simulink model "proc_control_node"  (R2020a)
settings: Solver=FixedStepAuto  StartTime=0.0  StopTime=inf  FixedStep=1/60  RelTol=1e-3
model workspace (MAT data in the model file):
  SL_ROS_VariableLengthArrays_MaxSizes.CommonInfo.ArrayTruncateAction = 'EmitWarning'
  SL_ROS_VariableLengthArrays_MaxSizes.MsgTypeMap = containers.Map
  SL_ROS_VariableLengthArrays_MaxSizes.MsgTypeMap.serialization.keys = {}
  SL_ROS_VariableLengthArrays_MaxSizes.MsgTypeMap.serialization.values = {}
  SL_ROS_VariableLengthArrays_MaxSizes.MsgTypeMap.serialization.uniformity = 0
  SL_ROS_VariableLengthArrays_MaxSizes.MsgTypeMap.serialization.keyType = 'char'
  SL_ROS_VariableLengthArrays_MaxSizes.MsgTypeMap.serialization.valueType = 'any'
undefined symbols (not defined in the file or in its folder): InitAUVPlant, InitController, mpc, physics, simulation
libraries: robotlib x21
settings Model: SimulationMode=accelerator  PauseTimes=1000  EnablePacing=on  Creator=Lamarre  LastModifiedBy=lamarre
settings OptimizationCC: EnhancedBackFolding=on  PassReuseOutputArgsAs=Individual arguments  ZeroExternalMemoryAtStartup=off  ZeroInternalMemoryAtStartup=off  MaxStackSize=64  OptimizeBlockOrder=speed  DifferentSizesBufferReuse=on  OptimizationCustomize=off  EfficientTunableParamExpr=on
settings DebuggingCC: ParameterTunabilityLossMsg=error  FcnCallInpInsideContextMsg=warning  UnderSpecifiedDimensionMsg=warning
settings HardwareCC: ProdBitPerPointer=32  ProdBitPerSizeT=32  ProdBitPerPtrDiffT=32  ProdLargestAtomicInteger=Long  ProdWordSize=32  ProdHWDeviceType=ARM Compatible->ARM 8
settings ModelReferenceCC: ModelReferenceNumInstancesAllowed=Single
settings SFSimCC: MATLABDynamicMemAlloc=off
settings RTWCC: SystemTargetFile=ert.tlc  HardwareBoard=Robot Operating System (ROS)  TemplateMakefile=ert_default_tmf  Toolchain=Catkin  BuildConfiguration=Faster Runs  TargetLang=C++
settings CodeAppCC: ForceParamTrailComments=on  IgnoreCustomStorageClasses=off  OperatorAnnotations=on  SimulinkDataObjDesc=on  SFDataObjDesc=on  InsertBlockDesc=on
settings ERTTargetCC: MultiInstanceERTCode=on  CodeInterfacePackaging=C++ class  SupportContinuousTime=on  SupportVariableSizeSignals=on  MultiInstanceErrorCode=Warning  RootIOFormat=Structure reference

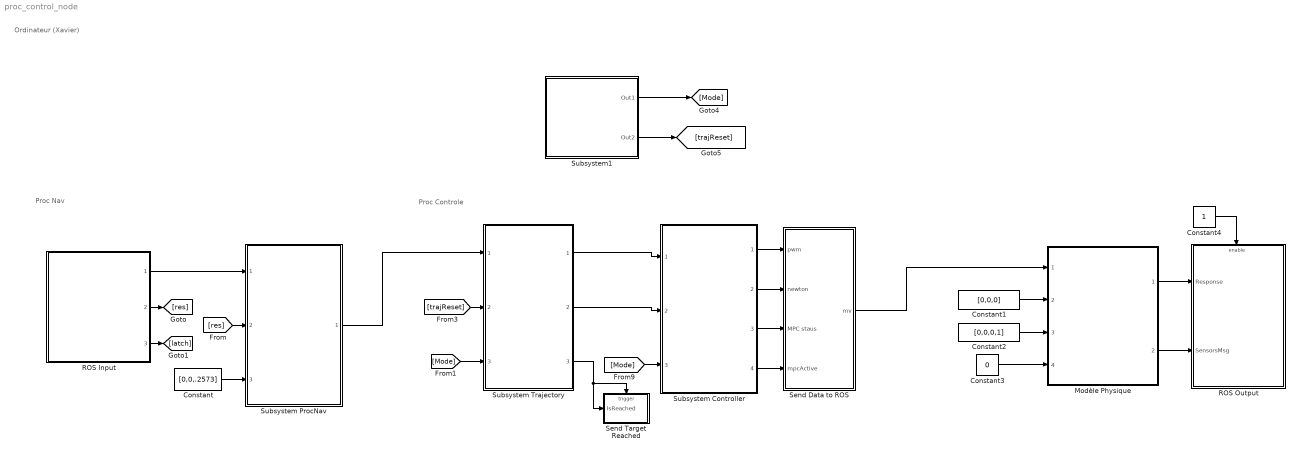
== system proc_control_node ==
  note: Proc Nav
  note: Proc Controle
  note: Ordinateur (Xavier)
  Constant : Constant  Value=[0,0,.2573]
  Constant1 : Constant  Value=[0,0,0]
  Constant2 : Constant  Value=[0,0,0,1]
  Constant3 : Constant  Value=0
  Constant4 : Constant
  Modèle Physique : Subsystem  InitFcn=InitAUVPlant;  ReferencedSubsystem=AUVPlant
  ROS Input : Subsystem  ReferencedSubsystem=proc_nav_ros_input
  ROS Output : Subsystem
  Send Data to ROS : Subsystem
  "Send Target Reached " : Subsystem
  Subsystem Controller : Subsystem  InitFcn=InitController;  ReferencedSubsystem=Controller
  Subsystem ProcNav : Subsystem  ReferencedSubsystem=ProcNav
  Subsystem Trajectory : Subsystem  InitFcn=|  ReferencedSubsystem=Trajectory
      | InitTrajectory
      | %trajec;
  Subsystem1 : Subsystem
  wires:
  Constant/1 -> Subsystem ProcNav/3
  ROS Input/1 -> Subsystem ProcNav/1
  ROS Input/2 -> [res]
  [res] -> Subsystem ProcNav/2
  ROS Input/3 -> [latch]
  [Mode] -> Subsystem Controller/3
  [Mode] -> Subsystem Trajectory/3
  Subsystem Trajectory/1 -> Subsystem Controller/1
  [trajReset] -> Subsystem Trajectory/2
  Subsystem Trajectory/3 -> "Send Target Reached "/1(IsReached), "Send Target Reached "/Trigger
  Subsystem ProcNav/1 -> Subsystem Trajectory/1
  Subsystem Trajectory/2 -> Subsystem Controller/2
  Subsystem1/2(Out2) -> [trajReset]
  Subsystem1/1(Out1) -> [Mode]
  Constant1/1 -> Modèle Physique/2
  Constant2/1 -> Modèle Physique/3
  Constant3/1 -> Modèle Physique/4
  Modèle Physique/1 -> ROS Output/1(Response)
  Modèle Physique/2 -> ROS Output/2(SensorsMsg)
  Constant4/1 -> ROS Output/Enable
  Subsystem Controller/1 -> Send Data to ROS/1(pwm)
  Subsystem Controller/2 -> Send Data to ROS/2(newton)
  Subsystem Controller/3 -> Send Data to ROS/3(MPC staus)
  Subsystem Controller/4 -> Send Data to ROS/4(mpcActive)
  Send Data to ROS/1(mv) -> Modèle Physique/1

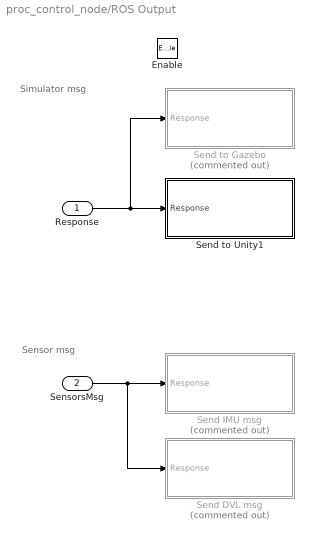
== system proc_control_node/ROS Output ==
  note: Sensor msg
  note: Simulator msg
  Response : Inport
  SensorsMsg : Inport  Port=2
  Enable : EnablePort
  Send DVL msg : Subsystem  Commented=on
  Send IMU msg : Subsystem  Commented=on
  Send to Gazebo : Subsystem  Commented=on  InitFcn=""
  Send to Unity1 : Subsystem
  wires:
  Response/1 -> Send to Unity1/1(Response), Send to Gazebo/1(Response)
  SensorsMsg/1 -> Send DVL msg/1(Response), Send IMU msg/1(Response)

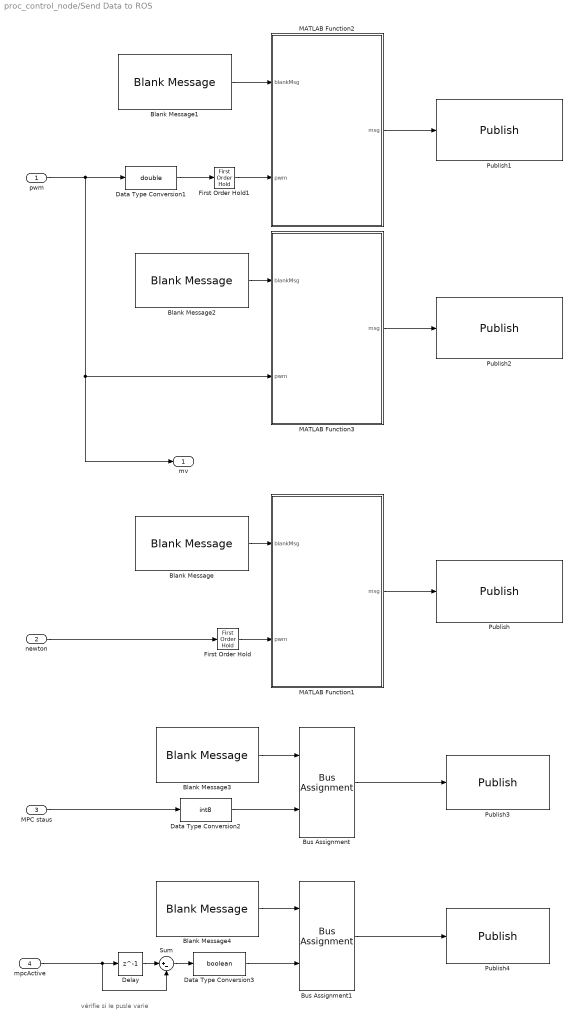
== system proc_control_node/Send Data to ROS ==
  note: vérifie si le pusle varie
  pwm : Inport
  newton : Inport  Port=2
  MPC staus : Inport  Port=3
  mpcActive : Inport  Port=4
  Blank Message : robotlib/Blank Message  messageClass=Message  entityType=std_msgs/Int8MultiArray  messageType=std_msgs/Int8MultiArray  SampleTime=inf
  Blank Message1 : robotlib/Blank Message  messageClass=Message  entityType=std_msgs/UInt16MultiArray  messageType=std_msgs/UInt16MultiArray  SampleTime=inf
  Blank Message2 : robotlib/Blank Message  messageClass=Message  entityType=std_msgs/UInt16MultiArray  messageType=std_msgs/UInt16MultiArray  SampleTime=inf
  Blank Message3 : robotlib/Blank Message  messageClass=Message  entityType=std_msgs/Int8  messageType=std_msgs/Int8  SampleTime=inf
  Blank Message4 : robotlib/Blank Message  messageClass=Message  entityType=std_msgs/Bool  messageType=std_msgs/Bool  SampleTime=-1
  Bus Assignment : BusAssignment  AssignedSignals=Data
  Bus Assignment1 : BusAssignment  AssignedSignals=Data
  Data Type Conversion1 : DataTypeConversion  OutDataTypeStr=double  RndMeth=Nearest
  Data Type Conversion2 : DataTypeConversion  OutDataTypeStr=int8  RndMeth=Nearest
  Data Type Conversion3 : DataTypeConversion  OutDataTypeStr=boolean  RndMeth=Nearest
  Delay : Delay  DelayLength=1  SampleTime=mpc.Ts
  First Order Hold : FirstOrderHold  ErrorTolerance=inf  AllowContinuousInput=on
  First Order Hold1 : FirstOrderHold  ErrorTolerance=inf  AllowContinuousInput=on
  MATLAB Function1 : MATLAB Function  TreatAsAtomicUnit=on  SystemSampleTime=1/30
  MATLAB Function2 : MATLAB Function  TreatAsAtomicUnit=on  SystemSampleTime=1/30
  MATLAB Function3 : MATLAB Function  TreatAsAtomicUnit=on
  Publish : robotlib/Publish  topicSource=Specify your own  topic=/telemetry/thruster_newton  messageType=std_msgs/Int8MultiArray  messageQueueLength=1
  Publish1 : robotlib/Publish  topicSource=Specify your own  topic=/telemetry/thruster_pwm  messageType=std_msgs/UInt16MultiArray  messageQueueLength=1
  Publish2 : robotlib/Publish  topicSource=Specify your own  topic=/provider_thruster/thruster_pwm  messageType=std_msgs/UInt16MultiArray  messageQueueLength=1
  Publish3 : robotlib/Publish  topicSource=Specify your own  topic=proc_control/mpc_status  messageType=std_msgs/Int8  messageQueueLength=1
  Publish4 : robotlib/Publish  topicSource=Specify your own  topic=proc_control/is_mpc_active  messageType=std_msgs/Bool  messageQueueLength=1
  Sum : Sum  Inputs=|+-
  mv : Outport
  wires:
  MATLAB Function1/1(msg) -> Publish/1
  Blank Message/1 -> MATLAB Function1/1(blankMsg)
  First Order Hold/1 -> MATLAB Function1/2(pwm)
  MATLAB Function2/1(msg) -> Publish1/1
  Blank Message1/1 -> MATLAB Function2/1(blankMsg)
  newton/1 -> First Order Hold/1
  Data Type Conversion1/1 -> First Order Hold1/1
  First Order Hold1/1 -> MATLAB Function2/2(pwm)
  MATLAB Function3/1(msg) -> Publish2/1
  pwm/1 -> mv/1, MATLAB Function3/2(pwm), Data Type Conversion1/1
  Blank Message2/1 -> MATLAB Function3/1(blankMsg)
  Blank Message3/1 -> Bus Assignment/1
  Bus Assignment/1 -> Publish3/1
  Data Type Conversion2/1 -> Bus Assignment/2
  MPC staus/1 -> Data Type Conversion2/1
  Data Type Conversion3/1 -> Bus Assignment1/2
  Bus Assignment1/1 -> Publish4/1
  Blank Message4/1 -> Bus Assignment1/1
  mpcActive/1 -> Delay/1, Sum/2
  Delay/1 -> Sum/1
  Sum/1 -> Data Type Conversion3/1

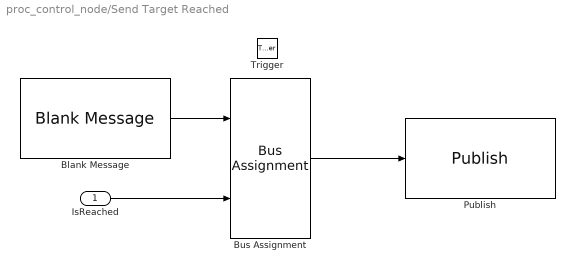
== system proc_control_node/Send Target Reached  ==
  IsReached : Inport
  Trigger : TriggerPort  TriggerType=either  VariantControl=Variant  PortDimensions=1
  Blank Message : robotlib/Blank Message  messageClass=Message  entityType=std_msgs/Bool  messageType=std_msgs/Bool  SampleTime=inf
  Bus Assignment : BusAssignment  AssignedSignals=Data
  Publish : robotlib/Publish  topicSource=Specify your own  topic=proc_control_matlab/target_reached  messageType=std_msgs/Bool  messageQueueLength=1
  wires:
  Blank Message/1 -> Bus Assignment/1
  IsReached/1 -> Bus Assignment/2
  Bus Assignment/1 -> Publish/1

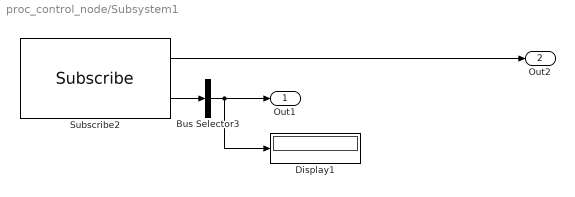
== system proc_control_node/Subsystem1 ==
  Bus Selector3 : BusSelector  OutputSignals=Data  OutputAsBus=on
  Display1 : Display
  Subscribe2 : robotlib/Subscribe  topicSource=Specify your own  topic=/proc_control/set_mode  messageType=std_msgs/UInt8  sampleTime=.25  messageQueueLength=1
  Out1 : Outport
  Out2 : Outport  Port=2
  wires:
  Subscribe2/1 -> Out2/1
  Bus Selector3/1 -> Display1/1, Out1/1
  Subscribe2/2 -> Bus Selector3/1

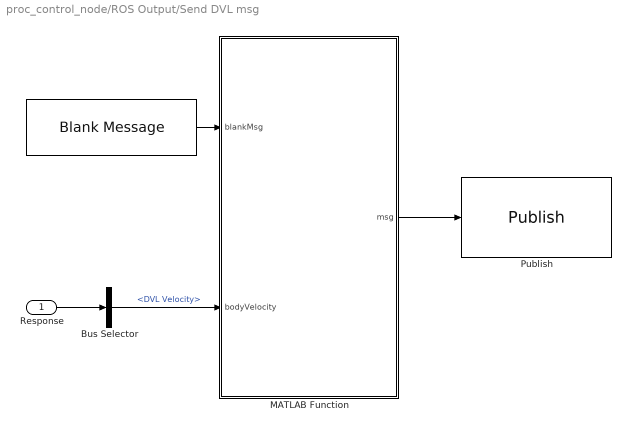
== system proc_control_node/ROS Output/Send DVL msg ==
  Response : Inport
  "   " : robotlib/Blank Message  messageClass=Message  entityType=sonia_common/BodyVelocityDVL  messageType=sonia_common/BodyVelocityDVL  SampleTime=1/60
  Bus Selector : BusSelector  OutputSignals=DVL Velocity
  MATLAB Function : MATLAB Function  TreatAsAtomicUnit=on  SystemSampleTime=1/60
  Publish : robotlib/Publish  topicSource=Specify your own  topic=/provider_dvl/dvl_velocity  messageType=sonia_common/BodyVelocityDVL  messageQueueLength=1
      link override SinkBlock: ROSTopic=/gazebo/set_model_state  ROSMessageType=gazebo_msgs/ModelState  SLBusName=SL_Bus_plant_gazebo_msgs_ModelState  ModelName=plant  BlockId=Pub_plant_206
  wires:
  Bus Selector/1 -> MATLAB Function/2(bodyVelocity)  "<DVL Velocity>"
  "   "/1 -> MATLAB Function/1(blankMsg)
  MATLAB Function/1(msg) -> Publish/1
  Response/1 -> Bus Selector/1

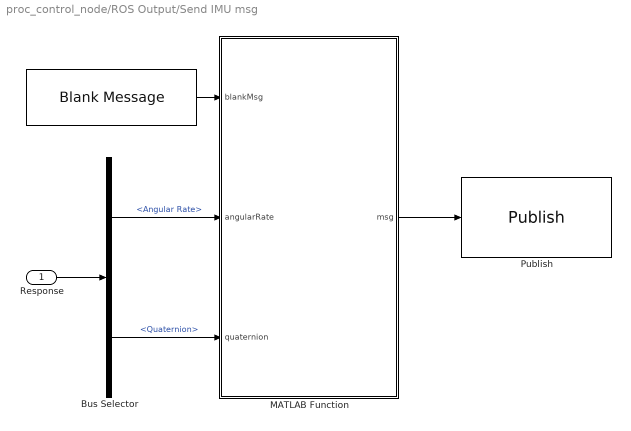
== system proc_control_node/ROS Output/Send IMU msg ==
  Response : Inport
  "   " : robotlib/Blank Message  messageClass=Message  entityType=sensor_msgs/Imu  messageType=sensor_msgs/Imu  SampleTime=1/60
  Bus Selector : BusSelector  OutputSignals=Angular Rate,Quaternion
  MATLAB Function : MATLAB Function  TreatAsAtomicUnit=on  SystemSampleTime=1/60
  Publish : robotlib/Publish  topicSource=Specify your own  topic=/provider_imu/imu_info  messageType=sensor_msgs/Imu  messageQueueLength=1
      link override SinkBlock: ROSTopic=/gazebo/set_model_state  ROSMessageType=gazebo_msgs/ModelState  SLBusName=SL_Bus_plant_gazebo_msgs_ModelState  ModelName=plant  BlockId=Pub_plant_206
  wires:
  Bus Selector/1 -> MATLAB Function/2(angularRate)  "<Angular Rate>"
  "   "/1 -> MATLAB Function/1(blankMsg)
  MATLAB Function/1(msg) -> Publish/1
  Response/1 -> Bus Selector/1
  Bus Selector/2 -> MATLAB Function/3(quaternion)  "<Quaternion>"

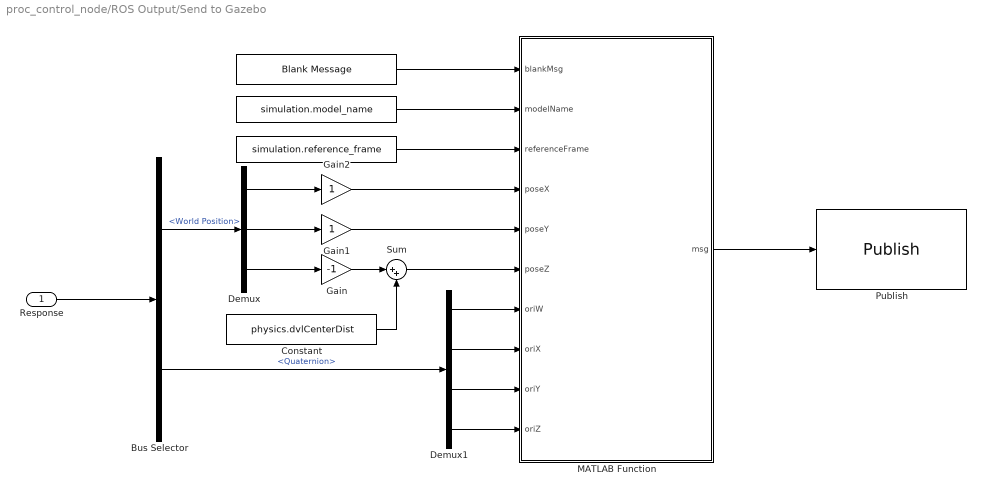
== system proc_control_node/ROS Output/Send to Gazebo ==
  Response : Inport
  " " : Constant  Value=simulation.model_name  VectorParams1D=off
  "  " : Constant  Value=simulation.reference_frame
  "   " : robotlib/Blank Message  messageClass=Message  entityType=gazebo_msgs/ModelState  messageType=gazebo_msgs/ModelState  SampleTime=1/60
  Bus Selector : BusSelector  OutputSignals=World Position,Quaternion
  Constant : Constant  Value=physics.dvlCenterDist
  Demux : Demux  Outputs=3
  Demux1 : Demux
  Gain : Gain  Gain=-1
  Gain1 : Gain
  Gain2 : Gain
  MATLAB Function : MATLAB Function  TreatAsAtomicUnit=on  SystemSampleTime=1/60
  Publish : robotlib/Publish  topicSource=Select from ROS network  topic=/gazebo/set_model_state  messageType=gazebo_msgs/ModelState  messageQueueLength=1
      link override SinkBlock: ROSTopic=/gazebo/set_model_state  ROSMessageType=gazebo_msgs/ModelState  SLBusName=SL_Bus_plant_gazebo_msgs_ModelState  ModelName=plant  BlockId=Pub_plant_206
  Sum : Sum  Inputs=|++
  wires:
  Bus Selector/1 -> Demux/1  "<World Position>"
  Demux/1 -> Gain2/1
  Demux/2 -> Gain1/1
  Demux/3 -> Gain/1
  "   "/1 -> MATLAB Function/1(blankMsg)
  "  "/1 -> MATLAB Function/3(referenceFrame)
  " "/1 -> MATLAB Function/2(modelName)
  Gain1/1 -> MATLAB Function/5(poseY)
  Bus Selector/2 -> Demux1/1  "<Quaternion>"
  Demux1/1 -> MATLAB Function/7(oriW)
  Demux1/2 -> MATLAB Function/8(oriX)
  Demux1/3 -> MATLAB Function/9(oriY)
  Demux1/4 -> MATLAB Function/10(oriZ)
  Gain2/1 -> MATLAB Function/4(poseX)
  MATLAB Function/1(msg) -> Publish/1
  Response/1 -> Bus Selector/1
  Gain/1 -> Sum/1
  Sum/1 -> MATLAB Function/6(poseZ)
  Constant/1 -> Sum/2

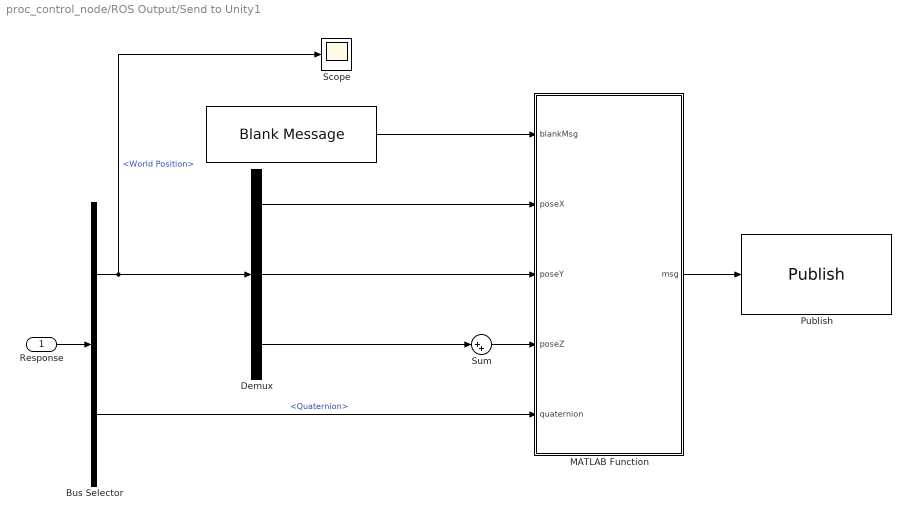
== system proc_control_node/ROS Output/Send to Unity1 ==
  Response : Inport
  "   " : robotlib/Blank Message  messageClass=Message  entityType=geometry_msgs/Pose  messageType=geometry_msgs/Pose  SampleTime=1/60
  Bus Selector : BusSelector  OutputSignals=World Position,Quaternion
  Demux : Demux  Outputs=3
  MATLAB Function : MATLAB Function  TreatAsAtomicUnit=on  SystemSampleTime=1/60
  Publish : robotlib/Publish  topicSource=Specify your own  topic=/pos_rot  messageType=geometry_msgs/Pose  messageQueueLength=1
      link override SinkBlock: ROSTopic=/gazebo/set_model_state  ROSMessageType=gazebo_msgs/ModelState  SLBusName=SL_Bus_plant_gazebo_msgs_ModelState  ModelName=plant  BlockId=Pub_plant_206
  Scope : Scope
  Sum : Sum  Inputs=|++
  wires:
  Bus Selector/1 -> Scope/1, Demux/1  "<World Position>"
  "   "/1 -> MATLAB Function/1(blankMsg)
  MATLAB Function/1(msg) -> Publish/1
  Response/1 -> Bus Selector/1
  Sum/1 -> MATLAB Function/4(poseZ)
  Demux/1 -> MATLAB Function/2(poseX)
  Demux/2 -> MATLAB Function/3(poseY)
  Demux/3 -> Sum/1
  Bus Selector/2 -> MATLAB Function/5(quaternion)  "<Quaternion>"

== matlab function proc_control_node/Send Data to ROS/MATLAB Function1 ==
  data: blankMsg input; pwm input; msg output Bus: SL_Bus_proc_control_node_std_msgs_Int8MultiArray
function msg = assignThrusterNewton(blankMsg, pwm)
msg = blankMsg;
msg.Data(1:8) = cast(pwm, 'int8');
msg.Data_SL_Info.CurrentLength = uint32(8);

== matlab function proc_control_node/ROS Output/Send DVL msg/MATLAB Function ==
  data: blankMsg input; bodyVelocity input; msg output Bus: SL_Bus_full_loop_sonia_common_BodyVelocityDVL
function msg = DVLmessage(blankMsg, bodyVelocity)
% assignStringInput - Assign a string in a ROS message to specified input string
%
% MSG = assignStringInput(blankMsg, STR) assigns the input string, STR, to
%  a string field in the ROS message, blankMsg, and outputs the updated
%  ROS message.
%
%  Inputs
%    blankMsg: A bus for a 'std_msgs/String' message. This is 
%        used to initialize the output.
%    str: An array of uint8 that will be assigned to the 'Data' field
%        in blankMsg. The entire array is assumed to be a valid sequence of
%        character ASCII values.
% 
%  Outputs:
%    msg: A bus for a 'std_msgs/String' message, with the 'Data'
%        field set to a string.

%   Copyright 2015 The MathWorks, Inc.
%#codegen

% Note: The datatype of 'msg' has been explicitly set to the appropriate 
% Simulink bus type ("Bus: SL_Bus_robotROSMessageUsageExample_std_msgs_String"). 
%
% If the model name is changed, the datatype needs to be changed as well:
%   1) Click "Edit Data" in the Editor toolstrip to open "Ports and Data Manager"
%   2) Select "msg". From the "Type" dropdown, select "--- Refresh data types ---"
%   3) Set datatype to "Bus: SL_Bus_<modelname>_std_msgs_String"
   
msg = blankMsg;


msg.XVelBtm = bodyVelocity(1);
msg.YVelBtm = bodyVelocity(2);
msg.ZVelBtm = bodyVelocity(3);

== matlab function proc_control_node/ROS Output/Send IMU msg/MATLAB Function ==
  data: blankMsg input; angularRate input; quaternion input; msg output Bus: SL_Bus_full_loop_sensor_msgs_Imu
function msg = IMUmessage(blankMsg, angularRate, quaternion)
% assignStringInput - Assign a string in a ROS message to specified input string
%
% MSG = assignStringInput(blankMsg, STR) assigns the input string, STR, to
%  a string field in the ROS message, blankMsg, and outputs the updated
%  ROS message.
%
%  Inputs
%    blankMsg: A bus for a 'std_msgs/String' message. This is 
%        used to initialize the output.
%    str: An array of uint8 that will be assigned to the 'Data' field
%        in blankMsg. The entire array is assumed to be a valid sequence of
%        character ASCII values.
% 
%  Outputs:
%    msg: A bus for a 'std_msgs/String' message, with the 'Data'
%        field set to a string.

%   Copyright 2015 The MathWorks, Inc.
%#codegen

% Note: The datatype of 'msg' has been explicitly set to the appropriate 
% Simulink bus type ("Bus: SL_Bus_robotROSMessageUsageExample_std_msgs_String"). 
%
% If the model name is changed, the datatype needs to be changed as well:
%   1) Click "Edit Data" in the Editor toolstrip to open "Ports and Data Manager"
%   2) Select "msg". From the "Type" dropdown, select "--- Refresh data types ---"
%   3) Set datatype to "Bus: SL_Bus_<modelname>_std_msgs_String"
   
msg = blankMsg;


msg.AngularVelocity.X = angularRate(1);
msg.AngularVelocity.Y = angularRate(2);
msg.AngularVelocity.Z = angularRate(3);

msg.Orientation.X = quaternion(2);
msg.Orientation.Y = quaternion(3);
msg.Orientation.Z = quaternion(4);
msg.Orientation.W = quaternion(1);

== matlab function proc_control_node/ROS Output/Send to Gazebo/MATLAB Function ==
  data: blankMsg input; msg output Bus: SL_Bus_proc_control_node_gazebo_msgs_ModelState; modelName input; referenceFrame input; poseX input; poseY input; poseZ input; oriW input; oriX input; oriY input; oriZ input
function msg = assignGazeboModelStateInput(blankMsg, modelName, referenceFrame, poseX, poseY, poseZ, oriW, oriX, oriY, oriZ)
% assignStringInput - Assign a string in a ROS message to specified input string
%
% MSG = assignStringInput(blankMsg, STR) assigns the input string, STR, to
%  a string field in the ROS message, blankMsg, and outputs the updated
%  ROS message.
%
%  Inputs
%    blankMsg: A bus for a 'std_msgs/String' message. This is 
%        used to initialize the output.
%    str: An array of uint8 that will be assigned to the 'Data' field
%        in blankMsg. The entire array is assumed to be a valid sequence of
%        character ASCII values.
% 
%  Outputs:
%    msg: A bus for a 'std_msgs/String' message, with the 'Data'
%        field set to a string.

%   Copyright 2015 The MathWorks, Inc.
%#codegen

% Note: The datatype of 'msg' has been explicitly set to the appropriate 
% Simulink bus type ("Bus: SL_Bus_robotROSMessageUsageExample_std_msgs_String"). 
%
% If the model name is changed, the datatype needs to be changed as well:
%   1) Click "Edit Data" in the Editor toolstrip to open "Ports and Data Manager"
%   2) Select "msg". From the "Type" dropdown, select "--- Refresh data types ---"
%   3) Set datatype to "Bus: SL_Bus_<modelname>_std_msgs_String"
   
msg = blankMsg;

strLength = length(modelName);
msg.ModelName(1:strLength) = modelName;
msg.ModelName_SL_Info.CurrentLength = uint32(strLength);

strLength = length(referenceFrame);
msg.ReferenceFrame(1:strLength) = referenceFrame;
msg.ReferenceFrame_SL_Info.CurrentLength = uint32(strLength);

msg.Pose.Position.X = poseX;
msg.Pose.Position.Y = poseY;
msg.Pose.Position.Z = poseZ;

msg.Pose.Orientation.X = oriX;
msg.Pose.Orientation.Y = oriY;
msg.Pose.Orientation.Z = oriZ;
msg.Pose.Orientation.W = oriW;

== matlab function proc_control_node/ROS Output/Send to Unity1/MATLAB Function ==
  data: blankMsg input; poseX input; poseY input; poseZ input; msg output Bus: SL_Bus_proc_control_node_geometry_msgs_Pose; quaternion input
function msg = assignUnityPoseRotInput(blankMsg, poseX, poseY, poseZ, quaternion)
% assignStringInput - Assign a string in a ROS message to specified input string
%
% MSG = assignStringInput(blankMsg, STR) assigns the input string, STR, to
%  a string field in the ROS message, blankMsg, and outputs the updated
%  ROS message.
%
%  Inputs
%    blankMsg: A bus for a 'std_msgs/String' message. This is 
%        used to initialize the output.
%    str: An array of uint8 that will be assigned to the 'Data' field
%        in blankMsg. The entire array is assumed to be a valid sequence of
%        character ASCII values.
% 
%  Outputs:
%    msg: A bus for a 'std_msgs/String' message, with the 'Data'
%        field set to a string.

%   Copyright 2015 The MathWorks, Inc.
%#codegen

% Note: The datatype of 'msg' has been explicitly set to the appropriate 
% Simulink bus type ("Bus: SL_Bus_robotROSMessageUsageExample_std_msgs_String"). 
%
% If the model name is changed, the datatype needs to be changed as well:
%   1) Click "Edit Data" in the Editor toolstrip to open "Ports and Data Manager"
%   2) Select "msg". From the "Type" dropdown, select "--- Refresh data types ---"
%   3) Set datatype to "Bus: SL_Bus_<modelname>_std_msgs_String"
   
msg = blankMsg;


msg.Position.X = poseX;
msg.Position.Y = poseY;
msg.Position.Z = poseZ;

msg.Orientation.X = quaternion(2);
msg.Orientation.Y = quaternion(3);
msg.Orientation.Z = quaternion(4);
msg.Orientation.W = quaternion(1);

== matlab function proc_control_node/Send Data to ROS/MATLAB Function2 ==
  data: blankMsg input; pwm input; msg output Bus: SL_Bus_proc_control_node_std_msgs_UInt16MultiArray
function msg = assignThrusterPwm(blankMsg, pwm)
msg = blankMsg;
msg.Data(1:8) = cast(pwm, 'uint16');
msg.Data_SL_Info.CurrentLength = uint32(8);

== matlab function proc_control_node/Send Data to ROS/MATLAB Function3 ==
  data: blankMsg input; pwm input; msg output Bus: SL_Bus_proc_control_node_std_msgs_UInt16MultiArray
function msg = assignThrusterPwm(blankMsg, pwm)
msg = blankMsg;
msg.Data(1:8) = cast(pwm, 'uint16');
msg.Data_SL_Info.CurrentLength = uint32(8);
